simulink subsystem "Bluetooth_Trayectoria"  (R2024b)
settings: Solver=VariableStepAuto  StartTime=0.0  StopTime=10.0  RelTol=1e-3
libraries: simulink x8
settings Model: Creator=Chenfu  LastModifiedBy=Chenfu

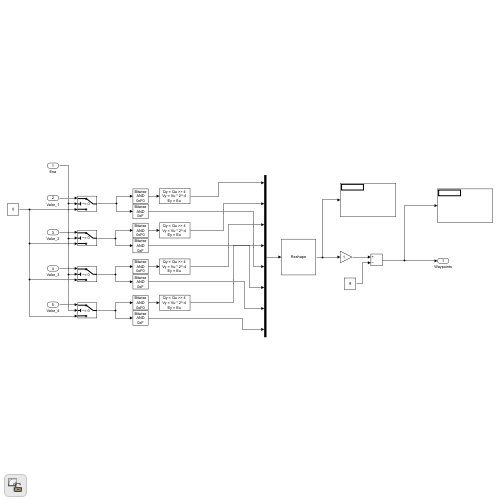
[thumbnail: Simulink's stored preview of the top-level diagram]
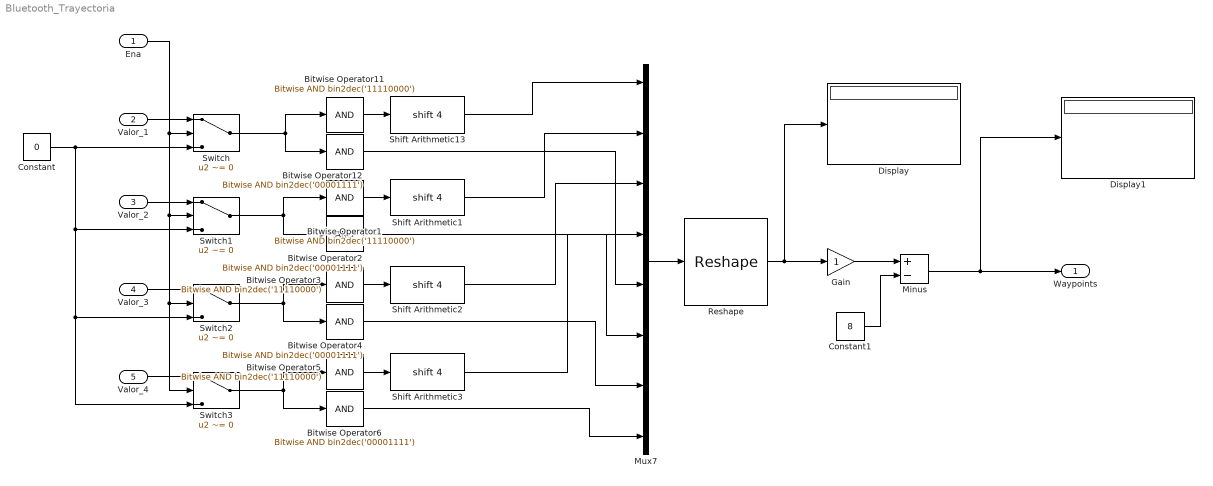
== system Bluetooth_Trayectoria ==
  Ena : Inport
  Valor_1 : Inport  Port=2
  Valor_2 : Inport  Port=3
  Valor_3 : Inport  Port=4
  Valor_4 : Inport  Port=5
  Bitwise Operator{1,3,5,11} (4 alike) : simulink/Logic and Bit Operations/Bitwise Operator  logicop=AND  UseBitMask=on  BitMask=bin2dec('11110000')  BitMaskRealWorld=Stored Integer
  Bitwise Operator{2,4,6,12} (4 alike) : simulink/Logic and Bit Operations/Bitwise Operator  logicop=AND  UseBitMask=on  BitMask=bin2dec('00001111')  BitMaskRealWorld=Stored Integer
  Constant : Constant  Value=0  OutDataTypeStr='uint8'
  Constant1 : Constant  Value=8
  Display : Display
  Display1 : Display
  Gain : Gain  OutDataTypeStr=double
  Minus : Sum  Inputs=+-
  Mux7 : Mux  Inputs=8
  Reshape : Reshape  OutputDimensionality=Customize  OutputDimensions=[4,2]
  Shift Arithmetic{1..3,13} (4 alike) : ArithShift  BitShiftNumber=4
  Switch{,1..3} (4 alike) : Switch  Criteria=u2 ~= 0  OutDataTypeStr=uint8  SaturateOnIntegerOverflow=off  InputSameDT=off
  Waypoints : Outport  OutDataTypeStr=double
  wires:
  Switch3/1 -> Bitwise Operator5/1, Bitwise Operator6/1
  Valor_1/1 -> Switch/1
  Ena/1 -> Switch/2, Switch1/2, Switch3/2, Switch2/2
  Constant/1 -> Switch1/3, Switch3/3, Switch2/3, Switch/3
  Valor_4/1 -> Switch3/1
  Valor_3/1 -> Switch2/1
  Valor_2/1 -> Switch1/1
  Switch2/1 -> Bitwise Operator4/1, Bitwise Operator3/1
  Switch/1 -> Bitwise Operator12/1, Bitwise Operator11/1
  Bitwise Operator11/1 -> Shift Arithmetic13/1
  Bitwise Operator1/1 -> Shift Arithmetic1/1
  Switch1/1 -> Bitwise Operator1/1, Bitwise Operator2/1
  Bitwise Operator3/1 -> Shift Arithmetic2/1
  Bitwise Operator5/1 -> Shift Arithmetic3/1
  Bitwise Operator6/1 -> Mux7/8
  Bitwise Operator4/1 -> Mux7/7
  Bitwise Operator2/1 -> Mux7/6
  Bitwise Operator12/1 -> Mux7/5
  Shift Arithmetic3/1 -> Mux7/4
  Shift Arithmetic2/1 -> Mux7/3
  Shift Arithmetic1/1 -> Mux7/2
  Shift Arithmetic13/1 -> Mux7/1
  Mux7/1 -> Reshape/1
  Reshape/1 -> Gain/1, Display/1
  Gain/1 -> Minus/1
  Minus/1 -> Waypoints/1, Display1/1
  Constant1/1 -> Minus/2
